simulink model "SLX2"  (R2019b)
settings: Solver=FixedStepDiscrete  StartTime=0.0  StopTime=10  FixedStep=0.01  RelTol=1e-3
settings Model: Creator=dingguoyu  LastModifiedBy=dingguoyu
settings OptimizationCC: LifeSpan=inf
settings DebuggingCC: ArithmeticOperatorsInVariantConditions=warning
settings SFSimCC: CustomCodeUndefinedFunction=UseInterfaceOnly
settings CodeAppCC: StateflowObjectComments=on

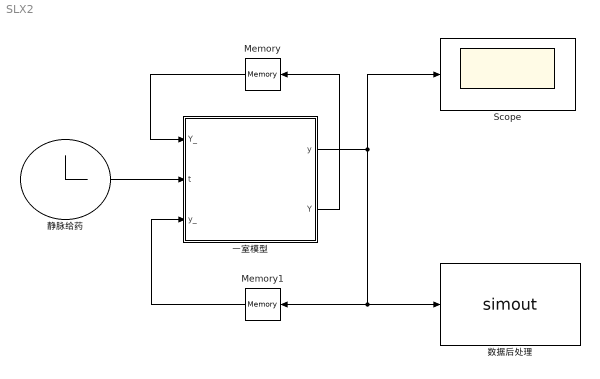
== system SLX2 ==
  Memory : Memory
  Memory1 : Memory
  Scope : Scope
  一室模型 : MATLAB Function  TreatAsAtomicUnit=on
  数据后处理 : ToWorkspace  VariableName=simout  SaveFormat=Timeseries  SampleTime=-1
      settings: Tag=血药浓度输出值
      mask Display: image('D:\AliWorkbenchData\Adobe Pre\b8dc54c6ecca6db850e038b25aba7cb3.jpeg'); % Use "Edit Image" on toolstrip to change.
  静脉给药 : Clock
      mask Display: image('D:\AliWorkbenchData\Adobe Pre\5e277f70cbeb5b57be28113bfa341aa9.jpeg'); % Use "Edit Image" on toolstrip to change.
  wires:
  静脉给药/1 -> 一室模型/2(t)
  一室模型/1(y) -> Scope/1, Memory1/1, 数据后处理/1
  Memory/1 -> 一室模型/1(Y_)
  一室模型/2(Y) -> Memory/1
  Memory1/1 -> 一室模型/3(y_)

== matlab function SLX2/一室模型 ==
  data: Y_ input; y output; Y output; t input; y_ input
function [y,Y]  = Interpolate3(Y_,t,y_)
%% 2022.6.15 by Ding Guo-yu & Li Qing-xin
%% input
c = 100; % 
k = 0.693; % 消除速率常数(Ke)
T = 1; % 给药间隔，τ
n=fix(t/T);
if t==0 
   % Y= c/(1-exp(-k*T)); % Cssmax 首剂量
     Y = c; % 正常给药
elseif t-T*n <= 0
     Y = c + Y_*exp(-k*(t-T*(n-1)));
else
     Y =Y_;   
end


%% output
if t <= T*(n+1)  
   y = Y*exp(-k*(t-T*n));
else
    y=-1;
end

end
